simulink model "miss_lab6"  (R2018a)
settings: Solver=ode45  StartTime=0.0  StopTime=15  MaxStep=2^-5  RelTol=1e-3
settings Model: Creator=Koala  LastModifiedBy=Koala

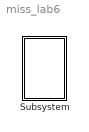
== system miss_lab6 ==
  Subsystem : Subsystem  mask{r0=1, fi0=90, g=9.81, m1=1, m2=2, k1=2, k2=1, M=1, R=0.001, fi10=80, fi20=150, l1=1, l2=2}

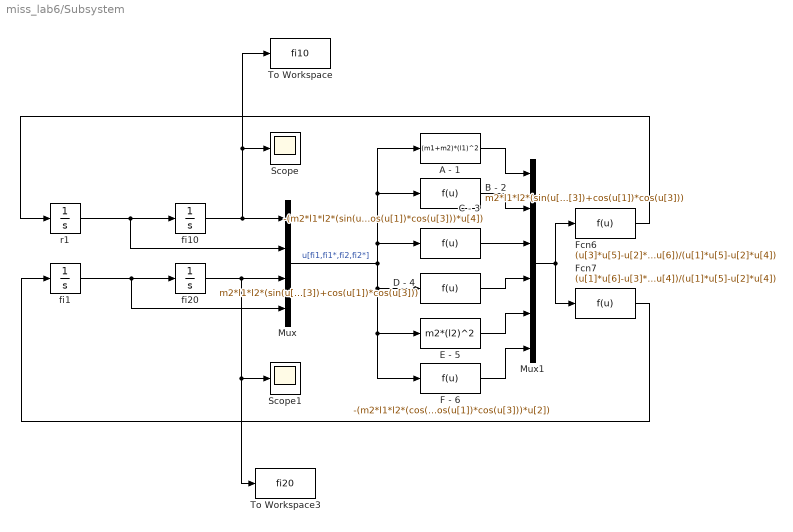
== system miss_lab6/Subsystem ==
  A - 1 : Fcn  Expr=(m1+m2)*(l1)^2
  B - 2 : Fcn  Expr=m2*l1*l2*(sin(u[1])*sin(u[3])+cos(u[1])*cos(u[3]))
  C - 3 : Fcn  Expr=-(m2*l1*l2*(sin(u[1])*cos(u[3])-cos(u[1])*sin(u[3]))*(u[4])^2 + (m1+m2)*g*(l1)*sin(u[1])+k1*(l1)^2*u[2]+k2*l1*l2*(sin(u[1])*sin(u[3])+cos(u[1])*cos(u[3]))*u[4])
  D - 4 : Fcn  Expr=m2*l1*l2*(sin(u[1])*sin(u[3])+cos(u[1])*cos(u[3]))
  E - 5 : Fcn  Expr=m2*(l2)^2
  F - 6 : Fcn  Expr=-(m2*l1*l2*(cos(u[1])*sin(u[3])-sin(u[1])*cos(u[3]))*(u[2])^2 + m2*g*l2*sin(u[3])+k2*(l2)^2*u[4]+k2*l1*l2*(sin(u[1])*sin(u[3])+cos(u[1])*cos(u[3]))*u[2])
  Fcn6 : Fcn  Expr=(u[3]*u[5]-u[2]*u[6])/(u[1]*u[5]-u[2]*u[4])
  Fcn7 : Fcn  Expr=(u[1]*u[6]-u[3]*u[4])/(u[1]*u[5]-u[2]*u[4])
  Mux : Mux
  Mux1 : Mux  Inputs=6
  Scope : Scope
  Scope1 : Scope
  To Workspace : ToWorkspace  VariableName=fi10  SampleTime=-1
  To Workspace3 : ToWorkspace  VariableName=fi20  SampleTime=-1
  fi1 : Integrator
  fi10 : Integrator  InitialCondition=fi10*pi/180
  fi20 : Integrator  InitialCondition=fi20*pi/180
  r1 : Integrator
  wires:
  fi10/1 -> To Workspace/1, Scope/1, Mux/1
  Fcn6/1 -> r1/1
  D - 4/1 -> Mux1/4
  F - 6/1 -> Mux1/6
  E - 5/1 -> Mux1/5
  fi20/1 -> To Workspace3/1, Scope1/1, Mux/3
  Mux/1 -> D - 4/1, F - 6/1, E - 5/1, A - 1/1, B - 2/1, C - 3/1  "u[fi1,fi1*,fi2,fi2*]"
  C - 3/1 -> Mux1/3
  B - 2/1 -> Mux1/2
  fi1/1 -> Mux/4, fi20/1
  Mux1/1 -> Fcn7/1, Fcn6/1
  A - 1/1 -> Mux1/1
  r1/1 -> Mux/2, fi10/1
  Fcn7/1 -> fi1/1
